simulink model "signal_tranmission"  (R2024b)
settings: Solver=ode45  StartTime=0.0  StopTime=10  FixedStep=0.000125  RelTol=1e-3
libraries: dspfdesign x500, commchan3 x1
(part 7 of 7)

== system signal_tranmission/SSB Modulator79/Balanced Modulator ==
  note: -S2(t)
  note: S1(t)
  note: -m(t)
  note: m(t)
  note: S2(t)
  note: S1(t)
  Input Signal : Inport
  Carrier Signal : Inport  Port=2
  -S2(t) : Product
  Add : Sum
  Add1 : Sum
  Add2 : Sum
  Constant : Constant
  Constant1 : Constant  Value=-1
  Constant2 : Constant
  Constant3 : Constant  Value=-1
  Product1 : Product
  S1(t) : Product
  S2(t) : Product
  DSBSC : Outport
  wires:
  Product1/1 -> Add1/1
  Add/1 -> S1(t)/1
  Constant3/1 -> -S2(t)/2
  Constant2/1 -> Add1/2
  S2(t)/1 -> -S2(t)/1
  Carrier Signal/1 -> S1(t)/2, S2(t)/1
  Constant/1 -> Add/2
  Add1/1 -> S2(t)/2
  Constant1/1 -> Product1/2
  -S2(t)/1 -> Add2/2
  S1(t)/1 -> Add2/1
  Input Signal/1 -> Product1/1, Add/1
  Add2/1 -> DSBSC/1

== system signal_tranmission/SSB Modulator8/Balanced Modulator ==
  note: -S2(t)
  note: S1(t)
  note: -m(t)
  note: m(t)
  note: S2(t)
  note: S1(t)
  Input Signal : Inport
  Carrier Signal : Inport  Port=2
  -S2(t) : Product
  Add : Sum
  Add1 : Sum
  Add2 : Sum
  Constant : Constant
  Constant1 : Constant  Value=-1
  Constant2 : Constant
  Constant3 : Constant  Value=-1
  Product1 : Product
  S1(t) : Product
  S2(t) : Product
  DSBSC : Outport
  wires:
  Product1/1 -> Add1/1
  Add/1 -> S1(t)/1
  Constant3/1 -> -S2(t)/2
  Constant2/1 -> Add1/2
  S2(t)/1 -> -S2(t)/1
  Carrier Signal/1 -> S1(t)/2, S2(t)/1
  Constant/1 -> Add/2
  Add1/1 -> S2(t)/2
  Constant1/1 -> Product1/2
  -S2(t)/1 -> Add2/2
  S1(t)/1 -> Add2/1
  Input Signal/1 -> Product1/1, Add/1
  Add2/1 -> DSBSC/1

== system signal_tranmission/SSB Modulator80/Balanced Modulator ==
  note: -S2(t)
  note: S1(t)
  note: -m(t)
  note: m(t)
  note: S2(t)
  note: S1(t)
  Input Signal : Inport
  Carrier Signal : Inport  Port=2
  -S2(t) : Product
  Add : Sum
  Add1 : Sum
  Add2 : Sum
  Constant : Constant
  Constant1 : Constant  Value=-1
  Constant2 : Constant
  Constant3 : Constant  Value=-1
  Product1 : Product
  S1(t) : Product
  S2(t) : Product
  DSBSC : Outport
  wires:
  Product1/1 -> Add1/1
  Add/1 -> S1(t)/1
  Constant3/1 -> -S2(t)/2
  Constant2/1 -> Add1/2
  S2(t)/1 -> -S2(t)/1
  Carrier Signal/1 -> S1(t)/2, S2(t)/1
  Constant/1 -> Add/2
  Add1/1 -> S2(t)/2
  Constant1/1 -> Product1/2
  -S2(t)/1 -> Add2/2
  S1(t)/1 -> Add2/1
  Input Signal/1 -> Product1/1, Add/1
  Add2/1 -> DSBSC/1

== system signal_tranmission/SSB Modulator81/Balanced Modulator ==
  note: -S2(t)
  note: S1(t)
  note: -m(t)
  note: m(t)
  note: S2(t)
  note: S1(t)
  Input Signal : Inport
  Carrier Signal : Inport  Port=2
  -S2(t) : Product
  Add : Sum
  Add1 : Sum
  Add2 : Sum
  Constant : Constant
  Constant1 : Constant  Value=-1
  Constant2 : Constant
  Constant3 : Constant  Value=-1
  Product1 : Product
  S1(t) : Product
  S2(t) : Product
  DSBSC : Outport
  wires:
  Product1/1 -> Add1/1
  Add/1 -> S1(t)/1
  Constant3/1 -> -S2(t)/2
  Constant2/1 -> Add1/2
  S2(t)/1 -> -S2(t)/1
  Carrier Signal/1 -> S1(t)/2, S2(t)/1
  Constant/1 -> Add/2
  Add1/1 -> S2(t)/2
  Constant1/1 -> Product1/2
  -S2(t)/1 -> Add2/2
  S1(t)/1 -> Add2/1
  Input Signal/1 -> Product1/1, Add/1
  Add2/1 -> DSBSC/1

== system signal_tranmission/SSB Modulator82/Balanced Modulator ==
  note: -S2(t)
  note: S1(t)
  note: -m(t)
  note: m(t)
  note: S2(t)
  note: S1(t)
  Input Signal : Inport
  Carrier Signal : Inport  Port=2
  -S2(t) : Product
  Add : Sum
  Add1 : Sum
  Add2 : Sum
  Constant : Constant
  Constant1 : Constant  Value=-1
  Constant2 : Constant
  Constant3 : Constant  Value=-1
  Product1 : Product
  S1(t) : Product
  S2(t) : Product
  DSBSC : Outport
  wires:
  Product1/1 -> Add1/1
  Add/1 -> S1(t)/1
  Constant3/1 -> -S2(t)/2
  Constant2/1 -> Add1/2
  S2(t)/1 -> -S2(t)/1
  Carrier Signal/1 -> S1(t)/2, S2(t)/1
  Constant/1 -> Add/2
  Add1/1 -> S2(t)/2
  Constant1/1 -> Product1/2
  -S2(t)/1 -> Add2/2
  S1(t)/1 -> Add2/1
  Input Signal/1 -> Product1/1, Add/1
  Add2/1 -> DSBSC/1

== system signal_tranmission/SSB Modulator83/Balanced Modulator ==
  note: -S2(t)
  note: S1(t)
  note: -m(t)
  note: m(t)
  note: S2(t)
  note: S1(t)
  Input Signal : Inport
  Carrier Signal : Inport  Port=2
  -S2(t) : Product
  Add : Sum
  Add1 : Sum
  Add2 : Sum
  Constant : Constant
  Constant1 : Constant  Value=-1
  Constant2 : Constant
  Constant3 : Constant  Value=-1
  Product1 : Product
  S1(t) : Product
  S2(t) : Product
  DSBSC : Outport
  wires:
  Product1/1 -> Add1/1
  Add/1 -> S1(t)/1
  Constant3/1 -> -S2(t)/2
  Constant2/1 -> Add1/2
  S2(t)/1 -> -S2(t)/1
  Carrier Signal/1 -> S1(t)/2, S2(t)/1
  Constant/1 -> Add/2
  Add1/1 -> S2(t)/2
  Constant1/1 -> Product1/2
  -S2(t)/1 -> Add2/2
  S1(t)/1 -> Add2/1
  Input Signal/1 -> Product1/1, Add/1
  Add2/1 -> DSBSC/1

== system signal_tranmission/SSB Modulator84/Balanced Modulator ==
  note: -S2(t)
  note: S1(t)
  note: -m(t)
  note: m(t)
  note: S2(t)
  note: S1(t)
  Input Signal : Inport
  Carrier Signal : Inport  Port=2
  -S2(t) : Product
  Add : Sum
  Add1 : Sum
  Add2 : Sum
  Constant : Constant
  Constant1 : Constant  Value=-1
  Constant2 : Constant
  Constant3 : Constant  Value=-1
  Product1 : Product
  S1(t) : Product
  S2(t) : Product
  DSBSC : Outport
  wires:
  Product1/1 -> Add1/1
  Add/1 -> S1(t)/1
  Constant3/1 -> -S2(t)/2
  Constant2/1 -> Add1/2
  S2(t)/1 -> -S2(t)/1
  Carrier Signal/1 -> S1(t)/2, S2(t)/1
  Constant/1 -> Add/2
  Add1/1 -> S2(t)/2
  Constant1/1 -> Product1/2
  -S2(t)/1 -> Add2/2
  S1(t)/1 -> Add2/1
  Input Signal/1 -> Product1/1, Add/1
  Add2/1 -> DSBSC/1

== system signal_tranmission/SSB Modulator85/Balanced Modulator ==
  note: -S2(t)
  note: S1(t)
  note: -m(t)
  note: m(t)
  note: S2(t)
  note: S1(t)
  Input Signal : Inport
  Carrier Signal : Inport  Port=2
  -S2(t) : Product
  Add : Sum
  Add1 : Sum
  Add2 : Sum
  Constant : Constant
  Constant1 : Constant  Value=-1
  Constant2 : Constant
  Constant3 : Constant  Value=-1
  Product1 : Product
  S1(t) : Product
  S2(t) : Product
  DSBSC : Outport
  wires:
  Product1/1 -> Add1/1
  Add/1 -> S1(t)/1
  Constant3/1 -> -S2(t)/2
  Constant2/1 -> Add1/2
  S2(t)/1 -> -S2(t)/1
  Carrier Signal/1 -> S1(t)/2, S2(t)/1
  Constant/1 -> Add/2
  Add1/1 -> S2(t)/2
  Constant1/1 -> Product1/2
  -S2(t)/1 -> Add2/2
  S1(t)/1 -> Add2/1
  Input Signal/1 -> Product1/1, Add/1
  Add2/1 -> DSBSC/1

== system signal_tranmission/SSB Modulator86/Balanced Modulator ==
  note: -S2(t)
  note: S1(t)
  note: -m(t)
  note: m(t)
  note: S2(t)
  note: S1(t)
  Input Signal : Inport
  Carrier Signal : Inport  Port=2
  -S2(t) : Product
  Add : Sum
  Add1 : Sum
  Add2 : Sum
  Constant : Constant
  Constant1 : Constant  Value=-1
  Constant2 : Constant
  Constant3 : Constant  Value=-1
  Product1 : Product
  S1(t) : Product
  S2(t) : Product
  DSBSC : Outport
  wires:
  Product1/1 -> Add1/1
  Add/1 -> S1(t)/1
  Constant3/1 -> -S2(t)/2
  Constant2/1 -> Add1/2
  S2(t)/1 -> -S2(t)/1
  Carrier Signal/1 -> S1(t)/2, S2(t)/1
  Constant/1 -> Add/2
  Add1/1 -> S2(t)/2
  Constant1/1 -> Product1/2
  -S2(t)/1 -> Add2/2
  S1(t)/1 -> Add2/1
  Input Signal/1 -> Product1/1, Add/1
  Add2/1 -> DSBSC/1

== system signal_tranmission/SSB Modulator87/Balanced Modulator ==
  note: -S2(t)
  note: S1(t)
  note: -m(t)
  note: m(t)
  note: S2(t)
  note: S1(t)
  Input Signal : Inport
  Carrier Signal : Inport  Port=2
  -S2(t) : Product
  Add : Sum
  Add1 : Sum
  Add2 : Sum
  Constant : Constant
  Constant1 : Constant  Value=-1
  Constant2 : Constant
  Constant3 : Constant  Value=-1
  Product1 : Product
  S1(t) : Product
  S2(t) : Product
  DSBSC : Outport
  wires:
  Product1/1 -> Add1/1
  Add/1 -> S1(t)/1
  Constant3/1 -> -S2(t)/2
  Constant2/1 -> Add1/2
  S2(t)/1 -> -S2(t)/1
  Carrier Signal/1 -> S1(t)/2, S2(t)/1
  Constant/1 -> Add/2
  Add1/1 -> S2(t)/2
  Constant1/1 -> Product1/2
  -S2(t)/1 -> Add2/2
  S1(t)/1 -> Add2/1
  Input Signal/1 -> Product1/1, Add/1
  Add2/1 -> DSBSC/1

== system signal_tranmission/SSB Modulator88/Balanced Modulator ==
  note: -S2(t)
  note: S1(t)
  note: -m(t)
  note: m(t)
  note: S2(t)
  note: S1(t)
  Input Signal : Inport
  Carrier Signal : Inport  Port=2
  -S2(t) : Product
  Add : Sum
  Add1 : Sum
  Add2 : Sum
  Constant : Constant
  Constant1 : Constant  Value=-1
  Constant2 : Constant
  Constant3 : Constant  Value=-1
  Product1 : Product
  S1(t) : Product
  S2(t) : Product
  DSBSC : Outport
  wires:
  Product1/1 -> Add1/1
  Add/1 -> S1(t)/1
  Constant3/1 -> -S2(t)/2
  Constant2/1 -> Add1/2
  S2(t)/1 -> -S2(t)/1
  Carrier Signal/1 -> S1(t)/2, S2(t)/1
  Constant/1 -> Add/2
  Add1/1 -> S2(t)/2
  Constant1/1 -> Product1/2
  -S2(t)/1 -> Add2/2
  S1(t)/1 -> Add2/1
  Input Signal/1 -> Product1/1, Add/1
  Add2/1 -> DSBSC/1

== system signal_tranmission/SSB Modulator89/Balanced Modulator ==
  note: -S2(t)
  note: S1(t)
  note: -m(t)
  note: m(t)
  note: S2(t)
  note: S1(t)
  Input Signal : Inport
  Carrier Signal : Inport  Port=2
  -S2(t) : Product
  Add : Sum
  Add1 : Sum
  Add2 : Sum
  Constant : Constant
  Constant1 : Constant  Value=-1
  Constant2 : Constant
  Constant3 : Constant  Value=-1
  Product1 : Product
  S1(t) : Product
  S2(t) : Product
  DSBSC : Outport
  wires:
  Product1/1 -> Add1/1
  Add/1 -> S1(t)/1
  Constant3/1 -> -S2(t)/2
  Constant2/1 -> Add1/2
  S2(t)/1 -> -S2(t)/1
  Carrier Signal/1 -> S1(t)/2, S2(t)/1
  Constant/1 -> Add/2
  Add1/1 -> S2(t)/2
  Constant1/1 -> Product1/2
  -S2(t)/1 -> Add2/2
  S1(t)/1 -> Add2/1
  Input Signal/1 -> Product1/1, Add/1
  Add2/1 -> DSBSC/1

== system signal_tranmission/SSB Modulator9/Balanced Modulator ==
  note: -S2(t)
  note: S1(t)
  note: -m(t)
  note: m(t)
  note: S2(t)
  note: S1(t)
  Input Signal : Inport
  Carrier Signal : Inport  Port=2
  -S2(t) : Product
  Add : Sum
  Add1 : Sum
  Add2 : Sum
  Constant : Constant
  Constant1 : Constant  Value=-1
  Constant2 : Constant
  Constant3 : Constant  Value=-1
  Product1 : Product
  S1(t) : Product
  S2(t) : Product
  DSBSC : Outport
  wires:
  Product1/1 -> Add1/1
  Add/1 -> S1(t)/1
  Constant3/1 -> -S2(t)/2
  Constant2/1 -> Add1/2
  S2(t)/1 -> -S2(t)/1
  Carrier Signal/1 -> S1(t)/2, S2(t)/1
  Constant/1 -> Add/2
  Add1/1 -> S2(t)/2
  Constant1/1 -> Product1/2
  -S2(t)/1 -> Add2/2
  S1(t)/1 -> Add2/1
  Input Signal/1 -> Product1/1, Add/1
  Add2/1 -> DSBSC/1

== system signal_tranmission/SSB Modulator90/Balanced Modulator ==
  note: -S2(t)
  note: S1(t)
  note: -m(t)
  note: m(t)
  note: S2(t)
  note: S1(t)
  Input Signal : Inport
  Carrier Signal : Inport  Port=2
  -S2(t) : Product
  Add : Sum
  Add1 : Sum
  Add2 : Sum
  Constant : Constant
  Constant1 : Constant  Value=-1
  Constant2 : Constant
  Constant3 : Constant  Value=-1
  Product1 : Product
  S1(t) : Product
  S2(t) : Product
  DSBSC : Outport
  wires:
  Product1/1 -> Add1/1
  Add/1 -> S1(t)/1
  Constant3/1 -> -S2(t)/2
  Constant2/1 -> Add1/2
  S2(t)/1 -> -S2(t)/1
  Carrier Signal/1 -> S1(t)/2, S2(t)/1
  Constant/1 -> Add/2
  Add1/1 -> S2(t)/2
  Constant1/1 -> Product1/2
  -S2(t)/1 -> Add2/2
  S1(t)/1 -> Add2/1
  Input Signal/1 -> Product1/1, Add/1
  Add2/1 -> DSBSC/1

== system signal_tranmission/SSB Modulator91/Balanced Modulator ==
  note: -S2(t)
  note: S1(t)
  note: -m(t)
  note: m(t)
  note: S2(t)
  note: S1(t)
  Input Signal : Inport
  Carrier Signal : Inport  Port=2
  -S2(t) : Product
  Add : Sum
  Add1 : Sum
  Add2 : Sum
  Constant : Constant
  Constant1 : Constant  Value=-1
  Constant2 : Constant
  Constant3 : Constant  Value=-1
  Product1 : Product
  S1(t) : Product
  S2(t) : Product
  DSBSC : Outport
  wires:
  Product1/1 -> Add1/1
  Add/1 -> S1(t)/1
  Constant3/1 -> -S2(t)/2
  Constant2/1 -> Add1/2
  S2(t)/1 -> -S2(t)/1
  Carrier Signal/1 -> S1(t)/2, S2(t)/1
  Constant/1 -> Add/2
  Add1/1 -> S2(t)/2
  Constant1/1 -> Product1/2
  -S2(t)/1 -> Add2/2
  S1(t)/1 -> Add2/1
  Input Signal/1 -> Product1/1, Add/1
  Add2/1 -> DSBSC/1

== system signal_tranmission/SSB Modulator92/Balanced Modulator ==
  note: -S2(t)
  note: S1(t)
  note: -m(t)
  note: m(t)
  note: S2(t)
  note: S1(t)
  Input Signal : Inport
  Carrier Signal : Inport  Port=2
  -S2(t) : Product
  Add : Sum
  Add1 : Sum
  Add2 : Sum
  Constant : Constant
  Constant1 : Constant  Value=-1
  Constant2 : Constant
  Constant3 : Constant  Value=-1
  Product1 : Product
  S1(t) : Product
  S2(t) : Product
  DSBSC : Outport
  wires:
  Product1/1 -> Add1/1
  Add/1 -> S1(t)/1
  Constant3/1 -> -S2(t)/2
  Constant2/1 -> Add1/2
  S2(t)/1 -> -S2(t)/1
  Carrier Signal/1 -> S1(t)/2, S2(t)/1
  Constant/1 -> Add/2
  Add1/1 -> S2(t)/2
  Constant1/1 -> Product1/2
  -S2(t)/1 -> Add2/2
  S1(t)/1 -> Add2/1
  Input Signal/1 -> Product1/1, Add/1
  Add2/1 -> DSBSC/1

== system signal_tranmission/SSB Modulator93/Balanced Modulator ==
  note: -S2(t)
  note: S1(t)
  note: -m(t)
  note: m(t)
  note: S2(t)
  note: S1(t)
  Input Signal : Inport
  Carrier Signal : Inport  Port=2
  -S2(t) : Product
  Add : Sum
  Add1 : Sum
  Add2 : Sum
  Constant : Constant
  Constant1 : Constant  Value=-1
  Constant2 : Constant
  Constant3 : Constant  Value=-1
  Product1 : Product
  S1(t) : Product
  S2(t) : Product
  DSBSC : Outport
  wires:
  Product1/1 -> Add1/1
  Add/1 -> S1(t)/1
  Constant3/1 -> -S2(t)/2
  Constant2/1 -> Add1/2
  S2(t)/1 -> -S2(t)/1
  Carrier Signal/1 -> S1(t)/2, S2(t)/1
  Constant/1 -> Add/2
  Add1/1 -> S2(t)/2
  Constant1/1 -> Product1/2
  -S2(t)/1 -> Add2/2
  S1(t)/1 -> Add2/1
  Input Signal/1 -> Product1/1, Add/1
  Add2/1 -> DSBSC/1

== system signal_tranmission/SSB Modulator94/Balanced Modulator ==
  note: -S2(t)
  note: S1(t)
  note: -m(t)
  note: m(t)
  note: S2(t)
  note: S1(t)
  Input Signal : Inport
  Carrier Signal : Inport  Port=2
  -S2(t) : Product
  Add : Sum
  Add1 : Sum
  Add2 : Sum
  Constant : Constant
  Constant1 : Constant  Value=-1
  Constant2 : Constant
  Constant3 : Constant  Value=-1
  Product1 : Product
  S1(t) : Product
  S2(t) : Product
  DSBSC : Outport
  wires:
  Product1/1 -> Add1/1
  Add/1 -> S1(t)/1
  Constant3/1 -> -S2(t)/2
  Constant2/1 -> Add1/2
  S2(t)/1 -> -S2(t)/1
  Carrier Signal/1 -> S1(t)/2, S2(t)/1
  Constant/1 -> Add/2
  Add1/1 -> S2(t)/2
  Constant1/1 -> Product1/2
  -S2(t)/1 -> Add2/2
  S1(t)/1 -> Add2/1
  Input Signal/1 -> Product1/1, Add/1
  Add2/1 -> DSBSC/1

== system signal_tranmission/SSB Modulator95/Balanced Modulator ==
  note: -S2(t)
  note: S1(t)
  note: -m(t)
  note: m(t)
  note: S2(t)
  note: S1(t)
  Input Signal : Inport
  Carrier Signal : Inport  Port=2
  -S2(t) : Product
  Add : Sum
  Add1 : Sum
  Add2 : Sum
  Constant : Constant
  Constant1 : Constant  Value=-1
  Constant2 : Constant
  Constant3 : Constant  Value=-1
  Product1 : Product
  S1(t) : Product
  S2(t) : Product
  DSBSC : Outport
  wires:
  Product1/1 -> Add1/1
  Add/1 -> S1(t)/1
  Constant3/1 -> -S2(t)/2
  Constant2/1 -> Add1/2
  S2(t)/1 -> -S2(t)/1
  Carrier Signal/1 -> S1(t)/2, S2(t)/1
  Constant/1 -> Add/2
  Add1/1 -> S2(t)/2
  Constant1/1 -> Product1/2
  -S2(t)/1 -> Add2/2
  S1(t)/1 -> Add2/1
  Input Signal/1 -> Product1/1, Add/1
  Add2/1 -> DSBSC/1

== system signal_tranmission/SSB Modulator96/Balanced Modulator ==
  note: -S2(t)
  note: S1(t)
  note: -m(t)
  note: m(t)
  note: S2(t)
  note: S1(t)
  Input Signal : Inport
  Carrier Signal : Inport  Port=2
  -S2(t) : Product
  Add : Sum
  Add1 : Sum
  Add2 : Sum
  Constant : Constant
  Constant1 : Constant  Value=-1
  Constant2 : Constant
  Constant3 : Constant  Value=-1
  Product1 : Product
  S1(t) : Product
  S2(t) : Product
  DSBSC : Outport
  wires:
  Product1/1 -> Add1/1
  Add/1 -> S1(t)/1
  Constant3/1 -> -S2(t)/2
  Constant2/1 -> Add1/2
  S2(t)/1 -> -S2(t)/1
  Carrier Signal/1 -> S1(t)/2, S2(t)/1
  Constant/1 -> Add/2
  Add1/1 -> S2(t)/2
  Constant1/1 -> Product1/2
  -S2(t)/1 -> Add2/2
  S1(t)/1 -> Add2/1
  Input Signal/1 -> Product1/1, Add/1
  Add2/1 -> DSBSC/1

== system signal_tranmission/SSB Modulator97/Balanced Modulator ==
  note: -S2(t)
  note: S1(t)
  note: -m(t)
  note: m(t)
  note: S2(t)
  note: S1(t)
  Input Signal : Inport
  Carrier Signal : Inport  Port=2
  -S2(t) : Product
  Add : Sum
  Add1 : Sum
  Add2 : Sum
  Constant : Constant
  Constant1 : Constant  Value=-1
  Constant2 : Constant
  Constant3 : Constant  Value=-1
  Product1 : Product
  S1(t) : Product
  S2(t) : Product
  DSBSC : Outport
  wires:
  Product1/1 -> Add1/1
  Add/1 -> S1(t)/1
  Constant3/1 -> -S2(t)/2
  Constant2/1 -> Add1/2
  S2(t)/1 -> -S2(t)/1
  Carrier Signal/1 -> S1(t)/2, S2(t)/1
  Constant/1 -> Add/2
  Add1/1 -> S2(t)/2
  Constant1/1 -> Product1/2
  -S2(t)/1 -> Add2/2
  S1(t)/1 -> Add2/1
  Input Signal/1 -> Product1/1, Add/1
  Add2/1 -> DSBSC/1

== system signal_tranmission/SSB Modulator98/Balanced Modulator ==
  note: -S2(t)
  note: S1(t)
  note: -m(t)
  note: m(t)
  note: S2(t)
  note: S1(t)
  Input Signal : Inport
  Carrier Signal : Inport  Port=2
  -S2(t) : Product
  Add : Sum
  Add1 : Sum
  Add2 : Sum
  Constant : Constant
  Constant1 : Constant  Value=-1
  Constant2 : Constant
  Constant3 : Constant  Value=-1
  Product1 : Product
  S1(t) : Product
  S2(t) : Product
  DSBSC : Outport
  wires:
  Product1/1 -> Add1/1
  Add/1 -> S1(t)/1
  Constant3/1 -> -S2(t)/2
  Constant2/1 -> Add1/2
  S2(t)/1 -> -S2(t)/1
  Carrier Signal/1 -> S1(t)/2, S2(t)/1
  Constant/1 -> Add/2
  Add1/1 -> S2(t)/2
  Constant1/1 -> Product1/2
  -S2(t)/1 -> Add2/2
  S1(t)/1 -> Add2/1
  Input Signal/1 -> Product1/1, Add/1
  Add2/1 -> DSBSC/1

== system signal_tranmission/SSB Modulator99/Balanced Modulator ==
  note: -S2(t)
  note: S1(t)
  note: -m(t)
  note: m(t)
  note: S2(t)
  note: S1(t)
  Input Signal : Inport
  Carrier Signal : Inport  Port=2
  -S2(t) : Product
  Add : Sum
  Add1 : Sum
  Add2 : Sum
  Constant : Constant
  Constant1 : Constant  Value=-1
  Constant2 : Constant
  Constant3 : Constant  Value=-1
  Product1 : Product
  S1(t) : Product
  S2(t) : Product
  DSBSC : Outport
  wires:
  Product1/1 -> Add1/1
  Add/1 -> S1(t)/1
  Constant3/1 -> -S2(t)/2
  Constant2/1 -> Add1/2
  S2(t)/1 -> -S2(t)/1
  Carrier Signal/1 -> S1(t)/2, S2(t)/1
  Constant/1 -> Add/2
  Add1/1 -> S2(t)/2
  Constant1/1 -> Product1/2
  -S2(t)/1 -> Add2/2
  S1(t)/1 -> Add2/1
  Input Signal/1 -> Product1/1, Add/1
  Add2/1 -> DSBSC/1
